simulink model "EGAS"  (R2025b)
settings: Solver=FixedStepAuto  StartTime=0.0  StopTime=5  RelTol=1e-3  EnableMultiTasking=on
model workspace (MAT data in the model file):
  Cs = 3
  J = 0.000245
  Kd = 0.03
  Ki = 0.2
  Kp = 2
  Ks = 0.2
  Ts = 0.1
  theta_eq = 0.523598775598
libraries: simulink x1
settings Model: Creator=vvpai9  LastModifiedBy=Pai
settings SolverCC: PositivePriorityOrder=on
settings OptimizationCC: EnhancedBackFolding=on  PassReuseOutputArgsAs=Individual arguments  ZeroExternalMemoryAtStartup=off  ZeroInternalMemoryAtStartup=off  MaxStackSize=200000  OptimizeBlockOrder=speed  DifferentSizesBufferReuse=on  OptimizationCustomize=off  EfficientTunableParamExpr=on
settings DebuggingCC: ParameterTunabilityLossMsg=error
settings HardwareCC: ProdBitPerLong=64.0  ProdLargestAtomicInteger=LongLong  ProdLargestAtomicFloat=Double  ProdLongLongMode=on  ProdHWDeviceType=ARM Compatible->ARM Cortex-A (64-bit)  UseEmbeddedCoderFeatures=off  UseSimulinkCoderFeatures=off
settings RTWCC: SystemTargetFile=ert.tlc  HardwareBoard=Raspberry Pi (64bit)  TLCOptions="-aInlineSetEventsForThisBaseRateFcn=TLC_FALSE -aSuppressMultiTaskScheduler=TLC_FALSE  -aRateBasedStepFcn=0"  GenCodeOnly=on  TemplateMakefile=ert_default_tmf  GenerateReport=on  Toolchain=GNU GCC Embedded Linux  BuildConfiguration=Faster Runs  LaunchReport=on  Description=Embedded Coder
settings CodeAppCC: ForceParamTrailComments=on  IgnoreCustomStorageClasses=off  OperatorAnnotations=on  SimulinkDataObjDesc=on  SFDataObjDesc=on  InsertBlockDesc=on
settings ERTTargetCC: ExtModeTransport=2.0  ExtModeStaticAlloc=on  ExtModeMexFile=ext_xcp  ExtModeIntrfLevel=Level2 - Open  InlinedParameterPlacement=Hierarchical  SupportNonInlinedSFcns=on  SupportVariableSizeSignals=on

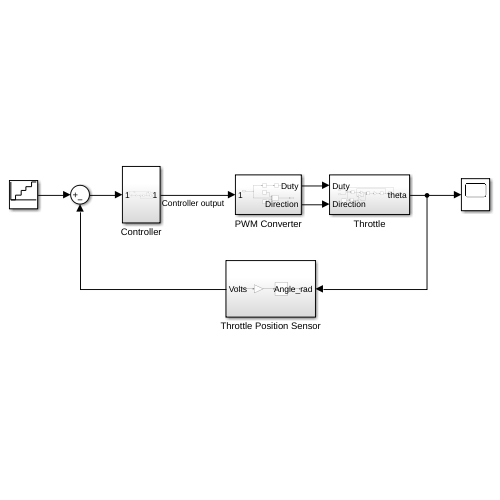
[thumbnail: Simulink's stored preview of the top-level diagram]
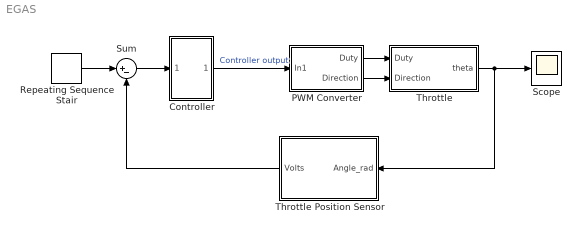
== system EGAS ==
  Controller : Subsystem
  PWM Converter : Subsystem
  Repeating Sequence Stair : simulink/Sources/Repeating Sequence Stair  OutValues=[0 1 2 3 4].'  tsamp=-1  OutMin=[]  OutMax=[]  OutDataTypeStr=double  OutputDataTypeScalingMode=double  OutDataType=fixdt(0,8)  ConRadixGroup=Best Precision: Vector-wise  OutScaling=2^-12
  Scope : Scope
      settings: ActiveDisplayYMinimum=-0.017544605677336962  ActiveDisplayYMaximum=0.21911278923821509
  Sum : Sum  Inputs=|+-
  Throttle : Subsystem
  Throttle Position Sensor : Subsystem
  wires:
  Controller/1(Out1) -> PWM Converter/1(In1)  "Controller output"
  PWM Converter/1(Duty) -> Throttle/1(Duty)
  PWM Converter/2(Direction) -> Throttle/2(Direction)
  Throttle/1(theta) -> Throttle Position Sensor/1(Angle_rad), Scope/1
  Sum/1 -> Controller/1(In1)
  Repeating Sequence Stair/1 -> Sum/1
  Throttle Position Sensor/1(Volts) -> Sum/2

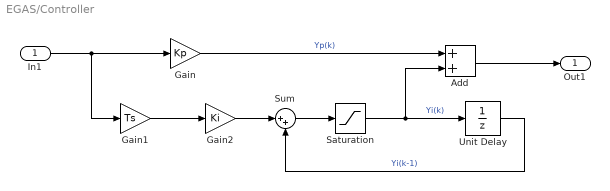
== system EGAS/Controller ==
  In1 : Inport
  Add : Sum
  Gain : Gain  Gain=Kp
  Gain1 : Gain  Gain=Ts
  Gain2 : Gain  Gain=Ki
  Saturation : Saturate  UpperLimit=1  LowerLimit=-1
  Sum : Sum  Inputs=|++
  Unit Delay : UnitDelay  SampleTime=-1  HasFrameUpgradeWarning=on
  Out1 : Outport
  wires:
  Gain1/1 -> Gain2/1
  Gain2/1 -> Sum/1
  Gain/1 -> Add/1  "Yp(k)"
  Unit Delay/1 -> Sum/2  "Yi(k-1)"
  Saturation/1 -> Unit Delay/1, Add/2  "Yi(k)"
  Sum/1 -> Saturation/1
  In1/1 -> Gain1/1, Gain/1
  Add/1 -> Out1/1

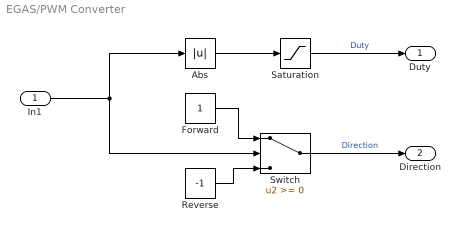
== system EGAS/PWM Converter ==
  In1 : Inport
  Abs : Abs  SaturateOnIntegerOverflow=off
  Forward : Constant
  Reverse : Constant  Value=-1
  Saturation : Saturate  UpperLimit=1  LowerLimit=0
  Switch : Switch  SaturateOnIntegerOverflow=off  InputSameDT=off
  Duty : Outport
  Direction : Outport  Port=2
  wires:
  Reverse/1 -> Switch/3
  Forward/1 -> Switch/1
  Abs/1 -> Saturation/1
  In1/1 -> Switch/2, Abs/1
  Saturation/1 -> Duty/1  "Duty"
  Switch/1 -> Direction/1  "Direction"

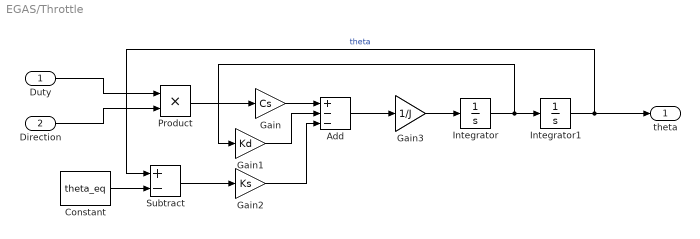
== system EGAS/Throttle ==
  Duty : Inport
  Direction : Inport  Port=2
  Add : Sum  Inputs=+--
  Constant : Constant  Value=theta_eq
  Gain : Gain  Gain=Cs
  Gain1 : Gain  Gain=Kd
  Gain2 : Gain  Gain=Ks
  Gain3 : Gain  Gain=1/J
  Integrator : Integrator
  Integrator1 : Integrator  InitialCondition=pi/6  LimitOutput=on  UpperSaturationLimit=pi/2  LowerSaturationLimit=0
  Product : Product
  Subtract : Sum  Inputs=+-
  theta : Outport
  wires:
  Subtract/1 -> Gain2/1
  Constant/1 -> Subtract/2
  Add/1 -> Gain3/1
  Gain/1 -> Add/1
  Gain2/1 -> Add/3
  Product/1 -> Gain/1
  Integrator/1 -> Integrator1/1, Gain1/1
  Gain1/1 -> Add/2
  Integrator1/1 -> theta/1, Subtract/1  "theta"
  Gain3/1 -> Integrator/1
  Direction/1 -> Product/2
  Duty/1 -> Product/1

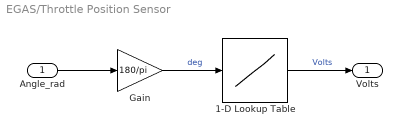
== system EGAS/Throttle Position Sensor ==
  Angle_rad : Inport
  1-D Lookup Table : Lookup_n-D  NumberOfTableDimensions=1  BreakpointsForDimension1=[0.5 4.5]  Table=[0 90]  InternalRulePriority=Speed  RndMeth=Simplest
  Gain : Gain  Gain=180/pi
  Volts : Outport
  wires:
  Gain/1 -> 1-D Lookup Table/1  "deg"
  1-D Lookup Table/1 -> Volts/1  "Volts"
  Angle_rad/1 -> Gain/1
